simulink model "Adaptive_LinearRegressionDynamics"  (R2024b)
settings: Solver=ode113  StartTime=0.0  StopTime=tf  RelTol=1e-3
values from neighbouring files (symbols this model uses):
  A_real = [0 1;-a0*(1+error) -a1*(1+error)]    [Model.m]
  ALambda = [0 1;-omega_n*omega_n -2*zeta*omega_n]    [LambdaDynamics.m]
  B_real = [0;1]    [Model.m]
  BLambda = [0;1]    [LambdaDynamics.m]
  C_omega1 = eye(2)    [LambdaDynamics.m]
  C_omega2 = eye(2)    [LambdaDynamics.m]
  C_real = C_nominal*(1+error)    [Model.m]
  C_x = eye(2)    [Model.m]
  D_x = [0;0]    [Model.m]
  DLambda = [0;0]    [LambdaDynamics.m]
  Gamma = [g1 0 0 0 ... (first row only)    [LambdaDynamics.m]
  omega_n = 10    [LambdaDynamics.m]
  u0 = 2    [Model.m]
  zeta = 0.7    [LambdaDynamics.m]
undefined symbols (not defined in the file or in its folder): IC, Noise
libraries: simulink x1
settings Model: Creator=perruquetti  LastModifiedBy=perruquetti
settings SolverCC: AlgebraicLoopSolver=TrustRegion
settings DataIOCC: ReturnWorkspaceOutputs=off
settings DebuggingCC: UnconnectedInputMsg=warning  UnconnectedOutputMsg=warning  UnconnectedLineMsg=warning  ArithmeticOperatorsInVariantConditions=warning
settings ModelReferenceCC: EnableRefExpFcnMdlSchedulingChecks=on
settings SFSimCC: SimUseLocalCustomCode=off  CustomCodeUndefinedFunction=UseInterfaceOnly
settings RTWCC: RTWUseLocalCustomCode=off  GPUComputeCapability=3.5  DLArmComputeVersion=19.05

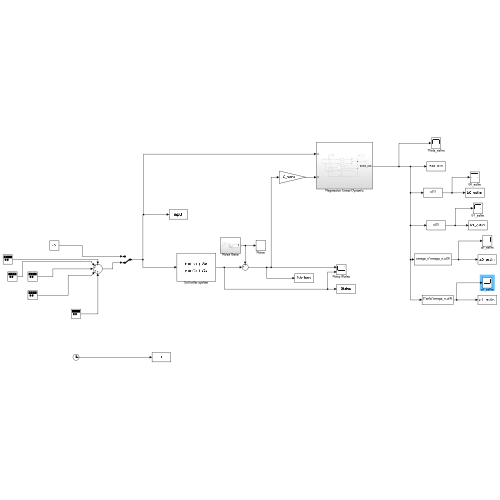
[thumbnail: Simulink's stored preview of the top-level diagram]
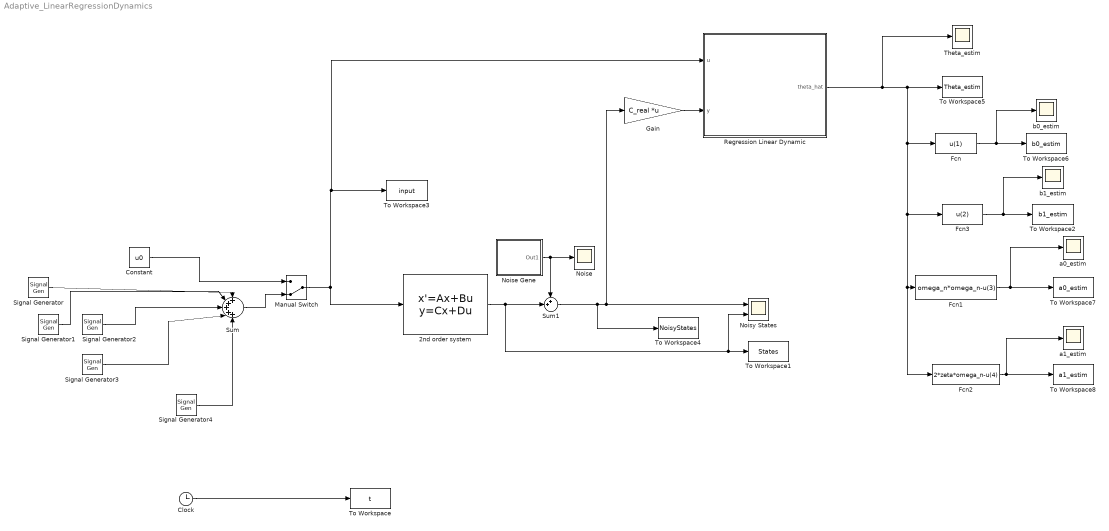
== system Adaptive_LinearRegressionDynamics ==
  2nd order system : StateSpace  A=A_real  B=B_real  C=C_x  D=D_x  InitialCondition=IC.state
  Clock : Clock
  Constant : Constant  Value=u0
  Fcn : Fcn  Expr=u(1)
  Fcn1 : Fcn  Expr=omega_n*omega_n-u(3)
  Fcn2 : Fcn  Expr=2*zeta*omega_n-u(4)
  Fcn3 : Fcn  Expr=u(2)
  Gain : Gain  Gain=C_real  Multiplication=Matrix(K*u)
  Manual Switch : ManualSwitch  CurrentSetting=0
  Noise : Scope
  Noise Gene : Subsystem
  Noisy States : Scope  NumInputPorts=2
  Regression Linear Dynamic : Subsystem
  Signal Generator : SignalGenerator  WaveForm=random  Amplitude=u0  Frequency=200  Units=rad/sec
  Signal Generator1 : SignalGenerator  WaveForm=random  Amplitude=u0  Frequency=100  Units=rad/sec
  Signal Generator2 : SignalGenerator  WaveForm=random  Amplitude=u0  Frequency=30  Units=rad/sec
  Signal Generator3 : SignalGenerator  WaveForm=random  Amplitude=u0  Frequency=10  Units=rad/sec
  Signal Generator4 : SignalGenerator  WaveForm=random  Amplitude=u0  Units=rad/sec
  Sum : Sum  Inputs=+++++
  Sum1 : Sum  Inputs=++|
  Theta_estim : Scope
  To Workspace : ToWorkspace  VariableName=t  SampleTime=-1
  To Workspace1 : ToWorkspace  VariableName=States  SampleTime=-1
  To Workspace2 : ToWorkspace  VariableName=b1_estim  SampleTime=-1
  To Workspace3 : ToWorkspace  VariableName=input  SampleTime=-1
  To Workspace4 : ToWorkspace  VariableName=NoisyStates  SampleTime=-1
  To Workspace5 : ToWorkspace  VariableName=Theta_estim  SampleTime=-1
  To Workspace6 : ToWorkspace  VariableName=b0_estim  SampleTime=-1
  To Workspace7 : ToWorkspace  VariableName=a0_estim  SampleTime=-1
  To Workspace8 : ToWorkspace  VariableName=a1_estim  SampleTime=-1
  a0_estim : Scope
  a1_estim : Scope
  b0_estim : Scope
  b1_estim : Scope
  wires:
  Manual Switch/1 -> 2nd order system/1, Regression Linear Dynamic/1(u), To Workspace3/1
  Gain/1 -> Regression Linear Dynamic/2(y)
  Constant/1 -> Manual Switch/1
  Clock/1 -> To Workspace/1
  2nd order system/1 -> Noisy States/2, To Workspace1/1, Sum1/2
  Sum1/1 -> Gain/1, Noisy States/1, To Workspace4/1
  Fcn/1 -> b0_estim/1, To Workspace6/1
  Fcn2/1 -> a1_estim/1, To Workspace8/1
  Fcn1/1 -> a0_estim/1, To Workspace7/1
  Fcn3/1 -> b1_estim/1, To Workspace2/1
  Regression Linear Dynamic/1(theta_hat) -> Theta_estim/1, Fcn/1, Fcn3/1, Fcn1/1, Fcn2/1, To Workspace5/1
  Noise Gene/1(Out1) -> Sum1/1, Noise/1
  Signal Generator/1 -> Sum/1
  Sum/1 -> Manual Switch/2
  Signal Generator4/1 -> Sum/5
  Signal Generator3/1 -> Sum/4
  Signal Generator2/1 -> Sum/3
  Signal Generator1/1 -> Sum/2

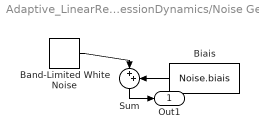
== system Adaptive_LinearRegressionDynamics/Noise Gene ==
  Band-Limited White Noise : simulink/Sources/Band-Limited White Noise  Cov=Noise.power  Ts=Noise.sampling  seed=Noise.seed
  Biais : Constant  Value=Noise.biais
  Sum : Sum  Inputs=|++
  Out1 : Outport
  wires:
  Sum/1 -> Out1/1
  Biais/1 -> Sum/2
  Band-Limited White Noise/1 -> Sum/1

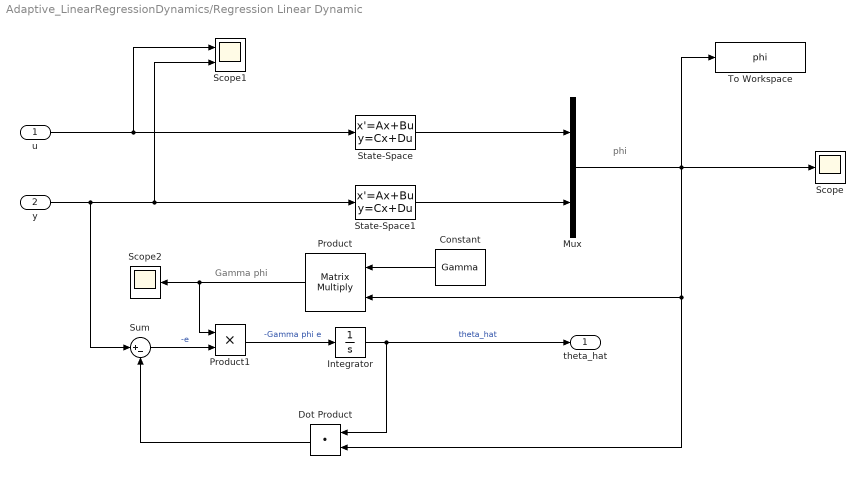
== system Adaptive_LinearRegressionDynamics/Regression Linear Dynamic ==
  note: Gamma phi
  note: phi
  u : Inport
  y : Inport  Port=2
  Constant : Constant  Value=Gamma
  Dot Product : DotProduct  OutDataTypeStr=Inherit: Inherit via internal rule
  Integrator : Integrator  InitialCondition=1
  Mux : Mux  Inputs=2
  Product : Product  Multiplication=Matrix(*)
  Product1 : Product
  Scope : Scope
  Scope1 : Scope  NumInputPorts=2
  Scope2 : Scope
  State-Space : StateSpace  A=ALambda  B=BLambda  C=C_omega1  D=DLambda  InitialCondition=IC.omega
  State-Space1 : StateSpace  A=ALambda  B=BLambda  C=C_omega2  D=DLambda  InitialCondition=IC.omega
  Sum : Sum  Inputs=|+-
  To Workspace : ToWorkspace  VariableName=phi  SampleTime=-1
  theta_hat : Outport  VectorParamsAs1DForOutWhenUnconnected=off
  wires:
  State-Space1/1 -> Mux/2
  Product1/1 -> Integrator/1  "-Gamma phi e"
  u/1 -> Scope1/1, State-Space/1
  State-Space/1 -> Mux/1
  Integrator/1 -> theta_hat/1, Dot Product/1  "theta_hat"
  Mux/1 -> To Workspace/1, Scope/1, Dot Product/2, Product/2
  Sum/1 -> Product1/2  "-e"
  Constant/1 -> Product/1
  y/1 -> Sum/1, Scope1/2, State-Space1/1
  Dot Product/1 -> Sum/2
  Product/1 -> Scope2/1, Product1/1
